simulink model "IEEE_39_case3"  (R2024b)
settings: Solver=ode3  StartTime=0  StopTime=40  FixedStep=Ts  MaxStep=1/60  RelTol=1e-3  AbsTol=1e-3  EnableMultiTasking=on
values from neighbouring files (symbols this model uses):
  c_f = c_f*Cb    [fun00_GFL_pu_2_normial.m]    (also in fun00_GFM_pu_2_normial.m)
  Dt = 0    [s02_case1.m]    (also in s02_case2.m; s03_case3.m; s03_case4.m; s03_case5.m)
  dw0_sm = 0    [s02_case1.m]    (also in s02_case2.m; s03_case3.m; s03_case4.m; s03_case5.m)
  Emax = 1.3    [s02_case1.m]    (also in s02_case2.m; s03_case3.m; s03_case4.m; s03_case5.m)
  Emin = 0.5    [s02_case1.m]    (also in s02_case2.m; s03_case3.m; s03_case4.m; s03_case5.m)
  Epss = 0.09    [s02_case1.m]    (also in s02_case2.m; s03_case3.m; s03_case4.m; s03_case5.m)
  fb = fn    (= 60)    [s02_case1.m]    (also in s02_case2.m; s03_case3.m; s03_case4.m; s03_case5.m)
  fn_sm = fn*ones(1,10)    [s02_case1.m]    (also in s02_case2.m; s03_case3.m; s03_case4.m; s03_case5.m)
  H_sm = [5,3.03,3.58,2.86,2.6,3.48,2.64,2.43,3.45,4.2]    [s02_case1.m]    (also in s02_case2.m; s03_case3.m; s03_case4.m; s03_case5.m)
  ia0_sm = 0    [s02_case1.m]    (also in s02_case2.m; s03_case3.m; s03_case4.m; s03_case5.m)
  ib0_sm = 0    [s02_case1.m]    (also in s02_case2.m; s03_case3.m; s03_case4.m; s03_case5.m)
  ic0_sm = 0    [s02_case1.m]    (also in s02_case2.m; s03_case3.m; s03_case4.m; s03_case5.m)
  Kd_sm = 0*ones(1,10)    [s02_case1.m]    (also in s02_case2.m; s03_case3.m; s03_case4.m; s03_case5.m)
  Ke = 1000    [s02_case1.m]    (also in s02_case2.m; s03_case3.m; s03_case4.m; s03_case5.m)
  ki_i = ki_i_pu*Vb_p_ph/Ib_p_ph    [fun00_GFL_pu_2_normial.m]    (also in fun00_GFM_pu_2_normial.m)
  ki_p = ki_p_pu/Sb*Ib_p_ph    [fun00_GFL_pu_2_normial.m]
  ki_pll = ki_pll/Vb_p_ph    [fun00_GFL_pu_2_normial.m]
  ki_q = ki_q_pu/Sb*Ib_p_ph    [fun00_GFL_pu_2_normial.m]
  kp_i = kp_i_pu*Vb_p_ph/Ib_p_ph    [fun00_GFL_pu_2_normial.m]    (also in fun00_GFM_pu_2_normial.m)
  kp_p = kp_p_pu/Sb*Ib_p_ph    [fun00_GFL_pu_2_normial.m]
  kp_pll = kp_pll/Vb_p_ph    [fun00_GFL_pu_2_normial.m]
  kp_q = kp_q_pu/Sb*Ib_p_ph    [fun00_GFL_pu_2_normial.m]
  Ks = 1    [s02_case1.m]    (also in s02_case2.m; s03_case3.m; s03_case4.m; s03_case5.m)
  l_f = l_f*Lb    [fun00_GFL_pu_2_normial.m]    (also in fun00_GFM_pu_2_normial.m)
  line = [     1	2	0.0035	0.0411	0.6987	0	100	345 ... (first row only)    [s02_case1.m]    (also in s02_case2.m; s03_case3.m; s03_case4.m; s03_case5.m)
  line_pu = line    [s02_case1.m]    (also in s02_case2.m; s03_case3.m; s03_case4.m; s03_case5.m)
  p = 1    [s02_case1.m]    (also in s02_case2.m; s03_case3.m; s03_case4.m; s03_case5.m)
  pha0_sm = 0    [s02_case1.m]    (also in s02_case2.m; s03_case3.m; s03_case4.m; s03_case5.m)
  phb0_sm = 0    [s02_case1.m]    (also in s02_case2.m; s03_case3.m; s03_case4.m; s03_case5.m)
  phc0_sm = 0    [s02_case1.m]    (also in s02_case2.m; s03_case3.m; s03_case4.m; s03_case5.m)
  Pn_sm = 1000*ones(1,num_gen)    [s02_case1.m]    (also in s02_case2.m; s03_case3.m; s03_case4.m; s03_case5.m)
  Pref_sm = [500 250 600 978 510 650 560 540 830 550]./Pn_sm    [s02_case1.m]    (also in s02_case2.m; s03_case3.m; s03_case4.m; s03_case5.m)
  pset = p_set_pu*Sb    [fun00_GFL_pu_2_normial.m]
  qset = q_set_pu*Sb    [fun00_GFL_pu_2_normial.m]
  R = 0.05    [s02_case1.m]    (also in s02_case2.m; s03_case3.m; s03_case4.m; s03_case5.m)
  r_f = r_f*Zb    [fun00_GFL_pu_2_normial.m]    (also in fun00_GFM_pu_2_normial.m)
  rs = 0.28    [s02_case1.m]    (also in s02_case2.m; s03_case3.m; s03_case4.m; s03_case5.m)
  Sb = 1000*10^6    (= 1000000000)    [s02_case1.m]    (also in s02_case2.m; s03_case3.m; s03_case4.m; s03_case5.m)
  T2 = 0.5    [s02_case1.m]    (also in s02_case2.m; s03_case3.m; s03_case4.m; s03_case5.m)
  T3 = 0.5    [s02_case1.m]    (also in s02_case2.m; s03_case3.m; s03_case4.m; s03_case5.m)
  t_gfl = 50    [s03_case3.m]    (also in s03_case4.m; s03_case5.m; s04_case6.m = 25; s04_case7.m = 25)
  t_gfm = 25    [s03_case3.m]    (also in s03_case4.m; s03_case5.m; s04_case6.m = 50; s04_case7.m = 50)
  t_s = 30    [s02_case1.m]    (also in s02_case2.m; s03_case3.m = 70; s03_case4.m = 70; s03_case5.m = 70)
  Te = 0.05    [s02_case1.m]    (also in s02_case2.m; s03_case3.m; s03_case4.m; s03_case5.m)
  Tfa = 3    [s02_case1.m]    (also in s02_case2.m; s03_case3.m; s03_case4.m; s03_case5.m)
  Tfb = 10    [s02_case1.m]    (also in s02_case2.m; s03_case3.m; s03_case4.m; s03_case5.m)
  theta0_sm = 0    [s02_case1.m]    (also in s02_case2.m; s03_case3.m; s03_case4.m; s03_case5.m)
  Ts = 1e-5    (= 1e-05)    [s02_case1.m]    (also in s02_case2.m; s03_case3.m; s03_case4.m; s03_case5.m)
  Ts1 = 0.76    [s02_case1.m]    (also in s02_case2.m; s03_case3.m; s03_case4.m; s03_case5.m)
  Ts2 = 0.1    [s02_case1.m]    (also in s02_case2.m; s03_case3.m; s03_case4.m; s03_case5.m)
  Ts3 = 0.76    [s02_case1.m]    (also in s02_case2.m; s03_case3.m; s03_case4.m; s03_case5.m)
  Ts4 = 0.1    [s02_case1.m]    (also in s02_case2.m; s03_case3.m; s03_case4.m; s03_case5.m)
  Ts5 = 10    [s02_case1.m]    (also in s02_case2.m; s03_case3.m; s03_case4.m; s03_case5.m)
  Un_sm = [345,22,22,22,22,22,22,22,345,22]    [s02_case1.m]    (also in s02_case2.m; s03_case3.m; s03_case4.m; s03_case5.m)
  Vb_gfm = 22*10^3    (= 22000)    [s02_case1.m]    (also in s02_case2.m; s03_case3.m; s03_case4.m; s03_case5.m)
  Vdc = 3*Vb_p_ph    [fun00_GFL_pu_2_normial.m]    (also in fun00_GFM_pu_2_normial.m)
  Vmax = 2    [s02_case1.m]    (also in s02_case2.m; s03_case3.m; s03_case4.m; s03_case5.m)
  Vmin = 0    [s02_case1.m]    (also in s02_case2.m; s03_case3.m; s03_case4.m; s03_case5.m)
  Vref_sm = 1*ones(1,10)    [s02_case1.m]    (also in s02_case2.m; s03_case3.m; s03_case4.m; s03_case5.m)
  w_b = fb*2*pi    [fun00_GFL_pu_2_normial.m]    (also in fun00_GFM_pu_2_normial.m; s02_case1.m = 376.991118431; s02_case2.m = 376.991118431; s03_case3.m = 376.991118431)
  wb = w_b    (= 376.991118431)    [s02_case1.m]    (also in s02_case2.m; s03_case3.m; s03_case4.m; s03_case5.m)
  xd = xd_t    (= 0.296)    [s02_case1.m]    (also in s02_case2.m; s03_case3.m; s03_case4.m; s03_case5.m)
undefined symbols (not defined in the file or in its folder): c_f_gfm, D1, D_p_gfm, D_p_gfm_s, D_q_gfm, Delta, DiscIntNeverNeededParam, Init, Init_GFL, J_gfm, Ka, Kf, ki_i_gfm, ki_pll_s, ki_vc_gfm, kp_i_gfm, kp_pll_s, kp_vc_gfm, l_f_gfm, P_set_gfm, Q_set_gfm, r_f_gfm, Ta, Tf, Vb, Vdc_gfm
libraries: spsThreePhaseVIMeasurementLib x76, spsabctodq0Lib x53, spsThreePhaseSeriesRLCBranchLib x52, slpidlib x50, spsThreePhaseParallelRLCLoadLib x20, spsThreePhaseTransformerTwoWindingsLib x12, spsdq0toabcLib x9, spsGroundLib x9, spsPowerPositiveSequenceLib x9, spsUniversalBridgeLib x9, spsDCVoltageSourceLib x9, spsFirstOrderFilterLib x1
(part 3 of 10)

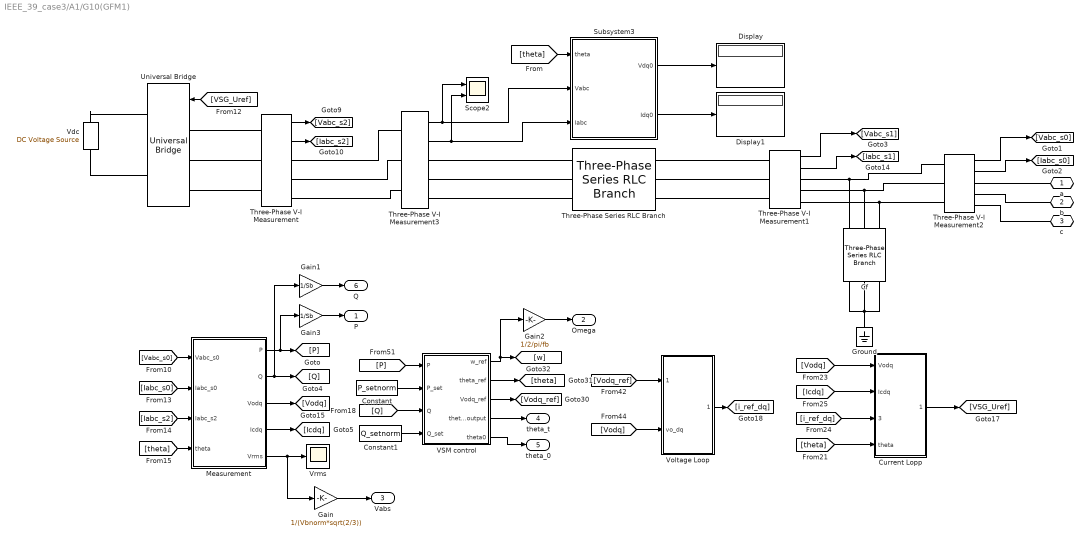
== system IEEE_39_case3/A1/G10(GFM1) ==
  Cf : spsThreePhaseSeriesRLCBranchLib/Three-Phase Series RLC Branch  LConnTagsString=A|B|C  RConnTagsString=A|B|C  BranchType=C  Resistance=0.1  Inductance=1e-3  Capacitance=RLCnorm(3)  Measurements=None
  Constant : Constant  Value=P_setnorm
  Constant1 : Constant  Value=Q_setnorm
  Current Lopp : Subsystem  mask{Current_P=Current_P, Current_I=Current_I}
      mask prompts: Current_P "Current Proportional Coefficient"; Current_I "Current Integral Coefficient"
  Display : Display
  Display1 : Display
  Gain : Gain  Gain=1/(Vbnorm*sqrt(2/3))
  Gain1 : Gain  Gain=1/Sb
  Gain2 : Gain  Gain=1/2/pi/fb
  Gain3 : Gain  Gain=1/Sb
  Ground : spsGroundLib/Ground  LConnTagsString=a
  Measurement : Subsystem
      mask DialogControl ParameterGroupVar Prompt: 参数
  Scope2 : Scope  NumInputPorts=2
  Subsystem3 : Subsystem
      mask DialogControl ParameterGroupVar Prompt: 参数
  Three-Phase Series RLC Branch : spsThreePhaseSeriesRLCBranchLib/Three-Phase Series RLC Branch  LConnTagsString=A|B|C  RConnTagsString=A|B|C  BranchType=RL  Resistance=RLCnorm(1)  Inductance=RLCnorm(2)  Capacitance=1e-6  Measurements=None
  Three-Phase V-I Measurement : spsThreePhaseVIMeasurementLib/Three-Phase V-I Measurement  VoltageMeasurement=phase-to-ground  SetLabelV=off  LabelV=Vabc_s2  Vpu=off  VpuLL=off  CurrentMeasurement=yes  SetLabelI=off  LabelI=Iabc_s2  Ipu=off  Pbase=Pnom  Vbase=Vnom  OutputType=Complex  PhasorSimulation=off  PSBequivalent=0
  Three-Phase V-I Measurement1 : spsThreePhaseVIMeasurementLib/Three-Phase V-I Measurement  VoltageMeasurement=phase-to-ground  SetLabelV=off  LabelV=Vabc_s1  Vpu=off  VpuLL=off  CurrentMeasurement=yes  SetLabelI=off  LabelI=Iabc_s1  Ipu=off  Pbase=Pnom  Vbase=Vnom  OutputType=Complex  PhasorSimulation=off  PSBequivalent=0
  Three-Phase V-I Measurement2 : spsThreePhaseVIMeasurementLib/Three-Phase V-I Measurement  VoltageMeasurement=phase-to-ground  SetLabelV=off  LabelV=Vabc_s0  Vpu=off  VpuLL=off  CurrentMeasurement=yes  SetLabelI=off  LabelI=Iabc_s0  Ipu=off  Pbase=Pnom  Vbase=Vnom  OutputType=Complex  PhasorSimulation=off  PSBequivalent=0
  Three-Phase V-I Measurement3 : spsThreePhaseVIMeasurementLib/Three-Phase V-I Measurement  VoltageMeasurement=phase-to-ground  SetLabelV=off  LabelV=Vabc_s2  Vpu=off  VpuLL=off  CurrentMeasurement=yes  SetLabelI=off  LabelI=Iabc_s2  Ipu=off  Pbase=Pnom  Vbase=Vnom  OutputType=Complex  PhasorSimulation=off  PSBequivalent=0
  Universal Bridge : spsUniversalBridgeLib/Universal Bridge  Arms=3  SnubberResistance=1e5  SnubberCapacitance=inf  Device=Average-model based VSC  Ron=1e-3  Lon=0  ForwardVoltages="[  0  0  ]"  ForwardVoltage=0  GTOparameters=[ 10e-6 , 20e-6 ]  IGBTparameters=[ 1e-6 , 2e-6 ]  Measurements=None  Measurements_2=None  converterType=Rectifier
  VSM control : Subsystem  mask{J=Jnorm, Dp=Dpnorm, Dq=Dqnorm}
      mask prompts: J "Inertia"; Dp "Damping"; Dq "Reactive Droop"
  Vdc : spsDCVoltageSourceLib/DC Voltage Source  Amplitude=Vdcnorm  Measurements=None
  Voltage Loop : Subsystem  mask{Voltage_P=Voltage_P, Voltage_I=Voltage_I}
      mask prompts: Voltage_P "Voltage Proportional Gain"; Voltage_I "Voltage Integral Gain"
  Vrms : Scope
  a : PMIOPort  Side=Right
  b : PMIOPort  Port=2  Side=Right
  c : PMIOPort  Port=3  Side=Right
  P : Outport
  Omega : Outport  Port=2
  Vabs : Outport  Port=3
  theta_t : Outport  Port=4
  theta_0 : Outport  Port=5
  Q : Outport  Port=6
  wires:
  [Vodq_ref] -> Voltage Loop/1(v_ref_dq)
  [Vodq] -> Voltage Loop/2(vo_dq)
  VSM control/2(theta_ref) -> [theta]
  Constant/1 -> VSM control/2(P_set)
  [P] -> VSM control/1(P)
  [Q] -> VSM control/3(Q)
  Three-Phase V-I Measurement1/2 -> [Iabc_s1]
  [VSG_Uref] -> Universal Bridge/1
  Subsystem3/1(Vdq0) -> Display/1
  Three-Phase V-I Measurement2/1 -> [Vabc_s0]
  Three-Phase V-I Measurement/2 -> [Iabc_s2]
  Three-Phase V-I Measurement3/2 -> Scope2/2, Subsystem3/3(Iabc)
  Subsystem3/2(Idq0) -> Display1/1
  Three-Phase V-I Measurement/1 -> [Vabc_s2]
  [theta] -> Subsystem3/1(theta)
  Three-Phase V-I Measurement2/2 -> [Iabc_s0]
  Three-Phase V-I Measurement3/1 -> Scope2/1, Subsystem3/2(Vabc)
  Three-Phase V-I Measurement1/1 -> [Vabc_s1]
  [Vabc_s0] -> Measurement/1(Vabc_s0)
  Measurement/5(Vrms) -> Gain/1, Vrms/1
  Measurement/2(Q) -> Gain1/1, [Q]
  Measurement/4(Icdq) -> [Icdq]
  Measurement/1(P) -> Gain3/1, [P]
  Measurement/3(Vodq) -> [Vodq]
  [theta] -> Measurement/4(theta)
  [Iabc_s2] -> Measurement/3(Iabc_s2)
  [Iabc_s0] -> Measurement/2(Iabc_s0)
  VSM control/3(Vodq_ref) -> [Vodq_ref]
  [Icdq] -> Current Lopp/2(Icdq)
  Current Lopp/1(VSG_Uref) -> [VSG_Uref]
  [Vodq] -> Current Lopp/1(Vodq)
  [theta] -> Current Lopp/4(theta)
  Voltage Loop/1(i_ref_dq) -> [i_ref_dq]
  [i_ref_dq] -> Current Lopp/3(i_ref_dq)
  Constant1/1 -> VSM control/4(Q_set)
  Gain/1 -> Vabs/1
  Gain3/1 -> P/1
  Gain2/1 -> Omega/1
  VSM control/1(w_ref) -> Gain2/1, [w]
  VSM control/4(theta_output) -> theta_t/1
  VSM control/5(theta0) -> theta_0/1
  Gain1/1 -> Q/1
  connections:
  Three-Phase V-I Measurement2/LConn1 -- Cf/LConn1 -- Three-Phase V-I Measurement1/RConn1
  Three-Phase V-I Measurement2/LConn2 -- Cf/LConn2 -- Three-Phase V-I Measurement1/RConn2
  Three-Phase V-I Measurement2/LConn3 -- Cf/LConn3 -- Three-Phase V-I Measurement1/RConn3
  Three-Phase V-I Measurement3/LConn1 -- Three-Phase V-I Measurement/RConn1
  Three-Phase V-I Measurement1/LConn3 -- Three-Phase Series RLC Branch/RConn3
  Three-Phase V-I Measurement2/RConn2 -- b/RConn1
  Three-Phase V-I Measurement/LConn3 -- Universal Bridge/LConn3
  Three-Phase V-I Measurement/LConn1 -- Universal Bridge/LConn1
  Vdc/RConn1 -- Universal Bridge/RConn1
  Three-Phase V-I Measurement2/RConn1 -- a/RConn1
  Three-Phase Series RLC Branch/LConn3 -- Three-Phase V-I Measurement3/RConn3
  Three-Phase V-I Measurement/LConn2 -- Universal Bridge/LConn2
  Three-Phase Series RLC Branch/LConn2 -- Three-Phase V-I Measurement3/RConn2
  Three-Phase V-I Measurement2/RConn3 -- c/RConn1
  Three-Phase V-I Measurement1/LConn1 -- Three-Phase Series RLC Branch/RConn1
  Three-Phase V-I Measurement3/RConn1 -- Three-Phase Series RLC Branch/LConn1
  Universal Bridge/RConn2 -- Vdc/LConn1
  Three-Phase V-I Measurement3/LConn3 -- Three-Phase V-I Measurement/RConn3
  Three-Phase V-I Measurement3/LConn2 -- Three-Phase V-I Measurement/RConn2
  Three-Phase V-I Measurement1/LConn2 -- Three-Phase Series RLC Branch/RConn2
  Cf/RConn3 -- Ground/LConn1 -- Cf/RConn2 -- Cf/RConn1

== system IEEE_39_case3/A1/G8(GFL4) ==
  Cf : spsThreePhaseSeriesRLCBranchLib/Three-Phase Series RLC Branch  LConnTagsString=A|B|C  RConnTagsString=A|B|C  BranchType=C  Resistance=0.1  Inductance=1e-3  Capacitance=RLC_Filter(3)  Measurements=None
  Constant : Constant  Value=Pref
  Constant1 : Constant  Value=Qref
  Display : Display
  Display1 : Display
  Gain : Gain  Gain=1/(Vnom*sqrt(2/3))
  Gain1 : Gain  Gain=1/Sb
  Gain2 : Gain  Gain=1/2/pi/fb
  Gain3 : Gain  Gain=1/Sb
  Ground : spsGroundLib/Ground  LConnTagsString=a
  Measurement : Subsystem
      mask DialogControl ParameterGroupVar Prompt: 参数
  PLL : Subsystem
      mask DialogControl ParameterGroupVar Prompt: 参数
  Subsystem3 : Subsystem
      mask DialogControl ParameterGroupVar Prompt: 参数
  Subsystem4 : Subsystem  mask{Voltage_P=Voltage_P, Voltage_I=Voltage_I, Current_P=Current_P, Current_I=Current_I, Power_P=Power_P, Power_I=Power_I, kf=kf}
      mask prompts: Voltage_P "Voltage Proportional Coefficient"; Voltage_I "Voltage Integral Coefficient"; Current_P "Current Proportional Coefficient"; Current_I "Current Integral Coefficient"; Power_P "Power Proportional Coefficient"; Power_I "Power Integral Coefficient"; kf "Feedforward Coeffcient"
      mask DialogControl ParameterGroupVar Prompt: Controller Parameter
  Three-Phase Series RLC Branch : spsThreePhaseSeriesRLCBranchLib/Three-Phase Series RLC Branch  LConnTagsString=A|B|C  RConnTagsString=A|B|C  BranchType=RL  Resistance=RLC_Filter(1)  Inductance=RLC_Filter(2)  Capacitance=1e-6  Measurements=None
  Three-Phase V-I Measurement : spsThreePhaseVIMeasurementLib/Three-Phase V-I Measurement  VoltageMeasurement=phase-to-ground  SetLabelV=off  LabelV=Vabc_s2  Vpu=off  VpuLL=off  CurrentMeasurement=yes  SetLabelI=off  LabelI=Iabc_s2  Ipu=off  Pbase=Pnom  Vbase=Vnom  OutputType=Complex  PhasorSimulation=off  PSBequivalent=0
  Three-Phase V-I Measurement1 : spsThreePhaseVIMeasurementLib/Three-Phase V-I Measurement  VoltageMeasurement=phase-to-ground  SetLabelV=off  LabelV=Vabc_s1  Vpu=off  VpuLL=off  CurrentMeasurement=yes  SetLabelI=off  LabelI=Iabc_s1  Ipu=off  Pbase=Pnom  Vbase=Vnom  OutputType=Complex  PhasorSimulation=off  PSBequivalent=0
  Three-Phase V-I Measurement2 : spsThreePhaseVIMeasurementLib/Three-Phase V-I Measurement  VoltageMeasurement=phase-to-ground  SetLabelV=off  LabelV=Vabc_s0  Vpu=off  VpuLL=off  CurrentMeasurement=yes  SetLabelI=off  LabelI=Iabc_s0  Ipu=off  Pbase=Pnom  Vbase=Vnom  OutputType=Complex  PhasorSimulation=off  PSBequivalent=0
  Three-Phase V-I Measurement3 : spsThreePhaseVIMeasurementLib/Three-Phase V-I Measurement  VoltageMeasurement=phase-to-ground  SetLabelV=off  LabelV=Vabc_s2  Vpu=off  VpuLL=off  CurrentMeasurement=yes  SetLabelI=off  LabelI=Iabc_s2  Ipu=off  Pbase=Pnom  Vbase=Vnom  OutputType=Complex  PhasorSimulation=off  PSBequivalent=0
  Universal Bridge : spsUniversalBridgeLib/Universal Bridge  Arms=3  SnubberResistance=1e5  SnubberCapacitance=inf  Device=Average-model based VSC  Ron=1e-3  Lon=0  ForwardVoltages="[  0  0  ]"  ForwardVoltage=0  GTOparameters=[ 10e-6 , 20e-6 ]  IGBTparameters=[ 1e-6 , 2e-6 ]  Measurements=None  Measurements_2=None  converterType=Rectifier
  Vdc : spsDCVoltageSourceLib/DC Voltage Source  Amplitude=Vdc_nom  Measurements=None
  Vrms : Scope
  a : PMIOPort  Side=Right
  b : PMIOPort  Port=2  Side=Right
  c : PMIOPort  Port=3  Side=Right
  P : Outport
  Omega : Outport  Port=2
  Vabs : Outport  Port=3
  theta_t : Outport  Port=4
  Q : Outport  Port=5
  theta_0 : Outport  Port=6
  wires:
  Measurement/5(Vrms) -> Gain/1, Vrms/1
  Measurement/2(Q) -> Gain1/1, [Q]
  Measurement/3(Vodq) -> [Vodq]
  Measurement/4(Icdq) -> [Icdq]
  [Vabc_s0] -> Measurement/1(Vabc_s0)
  [theta] -> Measurement/4(theta)
  [Iabc_s2] -> Measurement/3(Iabc_s2)
  [Iabc_s0] -> Measurement/2(Iabc_s0)
  [VSG_Uref] -> Universal Bridge/1
  [Vabc_s0] -> PLL/1(Vodq)
  Three-Phase V-I Measurement3/1 -> Subsystem3/1(Vabc)
  Three-Phase V-I Measurement3/2 -> Subsystem3/2(Iabc)
  Subsystem3/1(Vdq0) -> Display/1
  Subsystem3/2(Idq0) -> Display1/1
  PLL/2(theta) -> [theta]
  [Icdq] -> Subsystem4/2(Icdq)
  [Vodq] -> Subsystem4/1(Vodq)
  [theta] -> Subsystem4/3(theta)
  Subsystem4/1(VSG_Uref) -> [VSG_Uref]
  Three-Phase V-I Measurement/1 -> [Vabc_s2]
  Three-Phase V-I Measurement/2 -> [Iabc_s2]
  Three-Phase V-I Measurement2/1 -> [Vabc_s0]
  Three-Phase V-I Measurement2/2 -> [Iabc_s0]
  Three-Phase V-I Measurement1/2 -> [Iabc_s1]
  Three-Phase V-I Measurement1/1 -> [Vabc_s1]
  [P] -> Subsystem4/5(P)
  Constant/1 -> Subsystem4/4(pset)
  Constant1/1 -> Subsystem4/6(qset)
  [theta] -> Subsystem3/3(theta)
  Measurement/1(P) -> Gain3/1, [P]
  PLL/3(Omega) -> Gain2/1
  Gain/1 -> Vabs/1
  Gain2/1 -> Omega/1
  Gain3/1 -> P/1
  PLL/1(theta_GFL) -> theta_t/1
  Gain1/1 -> Q/1
  PLL/4(theta_0) -> theta_0/1
  [Q] -> Subsystem4/7(Q)
  connections:
  Three-Phase V-I Measurement2/LConn2 -- Cf/LConn2 -- Three-Phase V-I Measurement1/RConn2
  Three-Phase V-I Measurement2/LConn1 -- Cf/LConn1 -- Three-Phase V-I Measurement1/RConn1
  Three-Phase V-I Measurement2/LConn3 -- Cf/LConn3 -- Three-Phase V-I Measurement1/RConn3
  Three-Phase V-I Measurement1/LConn2 -- Three-Phase Series RLC Branch/RConn2
  Three-Phase V-I Measurement1/LConn1 -- Three-Phase Series RLC Branch/RConn1
  Universal Bridge/RConn2 -- Vdc/LConn1
  Vdc/RConn1 -- Universal Bridge/RConn1
  Three-Phase V-I Measurement/LConn3 -- Universal Bridge/LConn3
  Three-Phase V-I Measurement/LConn2 -- Universal Bridge/LConn2
  Three-Phase V-I Measurement/LConn1 -- Universal Bridge/LConn1
  Three-Phase V-I Measurement1/LConn3 -- Three-Phase Series RLC Branch/RConn3
  Three-Phase V-I Measurement2/RConn1 -- a/RConn1
  Three-Phase V-I Measurement2/RConn2 -- b/RConn1
  Three-Phase V-I Measurement2/RConn3 -- c/RConn1
  Three-Phase V-I Measurement3/RConn1 -- Three-Phase Series RLC Branch/LConn1
  Three-Phase Series RLC Branch/LConn2 -- Three-Phase V-I Measurement3/RConn2
  Three-Phase Series RLC Branch/LConn3 -- Three-Phase V-I Measurement3/RConn3
  Three-Phase V-I Measurement3/LConn1 -- Three-Phase V-I Measurement/RConn1
  Three-Phase V-I Measurement3/LConn2 -- Three-Phase V-I Measurement/RConn2
  Three-Phase V-I Measurement3/LConn3 -- Three-Phase V-I Measurement/RConn3
  Ground/LConn1 -- Cf/RConn2 -- Cf/RConn1 -- Cf/RConn3

== system IEEE_39_case3/A1/G9(GFL5) ==
  Cf : spsThreePhaseSeriesRLCBranchLib/Three-Phase Series RLC Branch  LConnTagsString=A|B|C  RConnTagsString=A|B|C  BranchType=C  Resistance=0.1  Inductance=1e-3  Capacitance=RLC_Filter(3)  Measurements=None
  Constant : Constant  Value=Pref
  Constant1 : Constant  Value=Qref
  Display : Display
  Display1 : Display
  Gain : Gain  Gain=1/(Vnom*sqrt(2/3))
  Gain1 : Gain  Gain=1/Sb
  Gain2 : Gain  Gain=1/2/pi/fb
  Gain3 : Gain  Gain=1/Sb
  Ground : spsGroundLib/Ground  LConnTagsString=a
  Measurement : Subsystem
      mask DialogControl ParameterGroupVar Prompt: 参数
  PLL : Subsystem
      mask DialogControl ParameterGroupVar Prompt: 参数
  Subsystem3 : Subsystem
      mask DialogControl ParameterGroupVar Prompt: 参数
  Subsystem4 : Subsystem  mask{Voltage_P=Voltage_P, Voltage_I=Voltage_I, Current_P=Current_P, Current_I=Current_I, Power_P=Power_P, Power_I=Power_I, kf=kf}
      mask prompts: Voltage_P "Voltage Proportional Coefficient"; Voltage_I "Voltage Integral Coefficient"; Current_P "Current Proportional Coefficient"; Current_I "Current Integral Coefficient"; Power_P "Power Proportional Coefficient"; Power_I "Power Integral Coefficient"; kf "Feedforward Coeffcient"
      mask DialogControl ParameterGroupVar Prompt: Controller Parameter
  Three-Phase Series RLC Branch : spsThreePhaseSeriesRLCBranchLib/Three-Phase Series RLC Branch  LConnTagsString=A|B|C  RConnTagsString=A|B|C  BranchType=RL  Resistance=RLC_Filter(1)  Inductance=RLC_Filter(2)  Capacitance=1e-6  Measurements=None
  Three-Phase V-I Measurement : spsThreePhaseVIMeasurementLib/Three-Phase V-I Measurement  VoltageMeasurement=phase-to-ground  SetLabelV=off  LabelV=Vabc_s2  Vpu=off  VpuLL=off  CurrentMeasurement=yes  SetLabelI=off  LabelI=Iabc_s2  Ipu=off  Pbase=Pnom  Vbase=Vnom  OutputType=Complex  PhasorSimulation=off  PSBequivalent=0
  Three-Phase V-I Measurement1 : spsThreePhaseVIMeasurementLib/Three-Phase V-I Measurement  VoltageMeasurement=phase-to-ground  SetLabelV=off  LabelV=Vabc_s1  Vpu=off  VpuLL=off  CurrentMeasurement=yes  SetLabelI=off  LabelI=Iabc_s1  Ipu=off  Pbase=Pnom  Vbase=Vnom  OutputType=Complex  PhasorSimulation=off  PSBequivalent=0
  Three-Phase V-I Measurement2 : spsThreePhaseVIMeasurementLib/Three-Phase V-I Measurement  VoltageMeasurement=phase-to-ground  SetLabelV=off  LabelV=Vabc_s0  Vpu=off  VpuLL=off  CurrentMeasurement=yes  SetLabelI=off  LabelI=Iabc_s0  Ipu=off  Pbase=Pnom  Vbase=Vnom  OutputType=Complex  PhasorSimulation=off  PSBequivalent=0
  Three-Phase V-I Measurement3 : spsThreePhaseVIMeasurementLib/Three-Phase V-I Measurement  VoltageMeasurement=phase-to-ground  SetLabelV=off  LabelV=Vabc_s2  Vpu=off  VpuLL=off  CurrentMeasurement=yes  SetLabelI=off  LabelI=Iabc_s2  Ipu=off  Pbase=Pnom  Vbase=Vnom  OutputType=Complex  PhasorSimulation=off  PSBequivalent=0
  Universal Bridge : spsUniversalBridgeLib/Universal Bridge  Arms=3  SnubberResistance=1e5  SnubberCapacitance=inf  Device=Average-model based VSC  Ron=1e-3  Lon=0  ForwardVoltages="[  0  0  ]"  ForwardVoltage=0  GTOparameters=[ 10e-6 , 20e-6 ]  IGBTparameters=[ 1e-6 , 2e-6 ]  Measurements=None  Measurements_2=None  converterType=Rectifier
  Vdc : spsDCVoltageSourceLib/DC Voltage Source  Amplitude=Vdc_nom  Measurements=None
  Vrms : Scope
  a : PMIOPort  Side=Right
  b : PMIOPort  Port=2  Side=Right
  c : PMIOPort  Port=3  Side=Right
  P : Outport
  Omega : Outport  Port=2
  Vabs : Outport  Port=3
  theta_t : Outport  Port=4
  Q : Outport  Port=5
  theta_0 : Outport  Port=6
  wires:
  Measurement/5(Vrms) -> Gain/1, Vrms/1
  Measurement/2(Q) -> Gain1/1, [Q]
  Measurement/3(Vodq) -> [Vodq]
  Measurement/4(Icdq) -> [Icdq]
  [Vabc_s0] -> Measurement/1(Vabc_s0)
  [theta] -> Measurement/4(theta)
  [Iabc_s2] -> Measurement/3(Iabc_s2)
  [Iabc_s0] -> Measurement/2(Iabc_s0)
  [VSG_Uref] -> Universal Bridge/1
  [Vabc_s0] -> PLL/1(Vodq)
  Three-Phase V-I Measurement3/1 -> Subsystem3/1(Vabc)
  Three-Phase V-I Measurement3/2 -> Subsystem3/2(Iabc)
  Subsystem3/1(Vdq0) -> Display/1
  Subsystem3/2(Idq0) -> Display1/1
  PLL/2(theta) -> [theta]
  [Icdq] -> Subsystem4/2(Icdq)
  [Vodq] -> Subsystem4/1(Vodq)
  [theta] -> Subsystem4/3(theta)
  Subsystem4/1(VSG_Uref) -> [VSG_Uref]
  Three-Phase V-I Measurement/1 -> [Vabc_s2]
  Three-Phase V-I Measurement/2 -> [Iabc_s2]
  Three-Phase V-I Measurement2/1 -> [Vabc_s0]
  Three-Phase V-I Measurement2/2 -> [Iabc_s0]
  Three-Phase V-I Measurement1/2 -> [Iabc_s1]
  Three-Phase V-I Measurement1/1 -> [Vabc_s1]
  [P] -> Subsystem4/5(P)
  Constant/1 -> Subsystem4/4(pset)
  Constant1/1 -> Subsystem4/6(qset)
  [theta] -> Subsystem3/3(theta)
  Measurement/1(P) -> Gain3/1, [P]
  PLL/3(Omega) -> Gain2/1
  Gain/1 -> Vabs/1
  Gain2/1 -> Omega/1
  Gain3/1 -> P/1
  PLL/1(theta_GFL) -> theta_t/1
  Gain1/1 -> Q/1
  PLL/4(theta_0) -> theta_0/1
  [Q] -> Subsystem4/7(Q)
  connections:
  Three-Phase V-I Measurement2/LConn2 -- Cf/LConn2 -- Three-Phase V-I Measurement1/RConn2
  Three-Phase V-I Measurement2/LConn1 -- Cf/LConn1 -- Three-Phase V-I Measurement1/RConn1
  Three-Phase V-I Measurement2/LConn3 -- Cf/LConn3 -- Three-Phase V-I Measurement1/RConn3
  Three-Phase V-I Measurement1/LConn2 -- Three-Phase Series RLC Branch/RConn2
  Three-Phase V-I Measurement1/LConn1 -- Three-Phase Series RLC Branch/RConn1
  Universal Bridge/RConn2 -- Vdc/LConn1
  Vdc/RConn1 -- Universal Bridge/RConn1
  Three-Phase V-I Measurement/LConn3 -- Universal Bridge/LConn3
  Three-Phase V-I Measurement/LConn2 -- Universal Bridge/LConn2
  Three-Phase V-I Measurement/LConn1 -- Universal Bridge/LConn1
  Three-Phase V-I Measurement1/LConn3 -- Three-Phase Series RLC Branch/RConn3
  Three-Phase V-I Measurement2/RConn1 -- a/RConn1
  Three-Phase V-I Measurement2/RConn2 -- b/RConn1
  Three-Phase V-I Measurement2/RConn3 -- c/RConn1
  Three-Phase V-I Measurement3/RConn1 -- Three-Phase Series RLC Branch/LConn1
  Three-Phase Series RLC Branch/LConn2 -- Three-Phase V-I Measurement3/RConn2
  Three-Phase Series RLC Branch/LConn3 -- Three-Phase V-I Measurement3/RConn3
  Three-Phase V-I Measurement3/LConn1 -- Three-Phase V-I Measurement/RConn1
  Three-Phase V-I Measurement3/LConn2 -- Three-Phase V-I Measurement/RConn2
  Three-Phase V-I Measurement3/LConn3 -- Three-Phase V-I Measurement/RConn3
  Ground/LConn1 -- Cf/RConn2 -- Cf/RConn1 -- Cf/RConn3

== system IEEE_39_case3/A2/G1(GFL1) ==
  Cf : spsThreePhaseSeriesRLCBranchLib/Three-Phase Series RLC Branch  LConnTagsString=A|B|C  RConnTagsString=A|B|C  BranchType=C  Resistance=0.1  Inductance=1e-3  Capacitance=RLC_Filter(3)  Measurements=None
  Constant : Constant  Value=Pref
  Constant1 : Constant  Value=Qref
  Display : Display
  Display1 : Display
  Gain : Gain  Gain=1/(Vnom*sqrt(2/3))
  Gain1 : Gain  Gain=1/Sb
  Gain2 : Gain  Gain=1/2/pi/fb
  Gain3 : Gain  Gain=1/Sb
  Ground : spsGroundLib/Ground  LConnTagsString=a
  Measurement : Subsystem
      mask DialogControl ParameterGroupVar Prompt: 参数
  PLL : Subsystem
      mask DialogControl ParameterGroupVar Prompt: 参数
  Subsystem3 : Subsystem
      mask DialogControl ParameterGroupVar Prompt: 参数
  Subsystem4 : Subsystem  mask{Voltage_P=Voltage_P, Voltage_I=Voltage_I, Current_P=Current_P, Current_I=Current_I, Power_P=Power_P, Power_I=Power_I, kf=kf}
      mask prompts: Voltage_P "Voltage Proportional Coefficient"; Voltage_I "Voltage Integral Coefficient"; Current_P "Current Proportional Coefficient"; Current_I "Current Integral Coefficient"; Power_P "Power Proportional Coefficient"; Power_I "Power Integral Coefficient"; kf "Feedforward Coeffcient"
      mask DialogControl ParameterGroupVar Prompt: Controller Parameter
  Three-Phase Series RLC Branch : spsThreePhaseSeriesRLCBranchLib/Three-Phase Series RLC Branch  LConnTagsString=A|B|C  RConnTagsString=A|B|C  BranchType=RL  Resistance=RLC_Filter(1)  Inductance=RLC_Filter(2)  Capacitance=1e-6  Measurements=None
  Three-Phase V-I Measurement : spsThreePhaseVIMeasurementLib/Three-Phase V-I Measurement  VoltageMeasurement=phase-to-ground  SetLabelV=off  LabelV=Vabc_s2  Vpu=off  VpuLL=off  CurrentMeasurement=yes  SetLabelI=off  LabelI=Iabc_s2  Ipu=off  Pbase=Pnom  Vbase=Vnom  OutputType=Complex  PhasorSimulation=off  PSBequivalent=0
  Three-Phase V-I Measurement1 : spsThreePhaseVIMeasurementLib/Three-Phase V-I Measurement  VoltageMeasurement=phase-to-ground  SetLabelV=off  LabelV=Vabc_s1  Vpu=off  VpuLL=off  CurrentMeasurement=yes  SetLabelI=off  LabelI=Iabc_s1  Ipu=off  Pbase=Pnom  Vbase=Vnom  OutputType=Complex  PhasorSimulation=off  PSBequivalent=0
  Three-Phase V-I Measurement2 : spsThreePhaseVIMeasurementLib/Three-Phase V-I Measurement  VoltageMeasurement=phase-to-ground  SetLabelV=off  LabelV=Vabc_s0  Vpu=off  VpuLL=off  CurrentMeasurement=yes  SetLabelI=off  LabelI=Iabc_s0  Ipu=off  Pbase=Pnom  Vbase=Vnom  OutputType=Complex  PhasorSimulation=off  PSBequivalent=0
  Three-Phase V-I Measurement3 : spsThreePhaseVIMeasurementLib/Three-Phase V-I Measurement  VoltageMeasurement=phase-to-ground  SetLabelV=off  LabelV=Vabc_s2  Vpu=off  VpuLL=off  CurrentMeasurement=yes  SetLabelI=off  LabelI=Iabc_s2  Ipu=off  Pbase=Pnom  Vbase=Vnom  OutputType=Complex  PhasorSimulation=off  PSBequivalent=0
  Universal Bridge : spsUniversalBridgeLib/Universal Bridge  Arms=3  SnubberResistance=1e5  SnubberCapacitance=inf  Device=Average-model based VSC  Ron=1e-3  Lon=0  ForwardVoltages="[  0  0  ]"  ForwardVoltage=0  GTOparameters=[ 10e-6 , 20e-6 ]  IGBTparameters=[ 1e-6 , 2e-6 ]  Measurements=None  Measurements_2=None  converterType=Rectifier
  Vdc : spsDCVoltageSourceLib/DC Voltage Source  Amplitude=Vdc_nom  Measurements=None
  Vrms : Scope
  a : PMIOPort  Side=Right
  b : PMIOPort  Port=2  Side=Right
  c : PMIOPort  Port=3  Side=Right
  P : Outport
  Omega : Outport  Port=2
  Vabs : Outport  Port=3
  theta_t : Outport  Port=4
  Q : Outport  Port=5
  theta_0 : Outport  Port=6
  wires:
  Measurement/5(Vrms) -> Gain/1, Vrms/1
  Measurement/2(Q) -> Gain1/1, [Q]
  Measurement/3(Vodq) -> [Vodq]
  Measurement/4(Icdq) -> [Icdq]
  [Vabc_s0] -> Measurement/1(Vabc_s0)
  [theta] -> Measurement/4(theta)
  [Iabc_s2] -> Measurement/3(Iabc_s2)
  [Iabc_s0] -> Measurement/2(Iabc_s0)
  [VSG_Uref] -> Universal Bridge/1
  [Vabc_s0] -> PLL/1(Vodq)
  Three-Phase V-I Measurement3/1 -> Subsystem3/1(Vabc)
  Three-Phase V-I Measurement3/2 -> Subsystem3/2(Iabc)
  Subsystem3/1(Vdq0) -> Display/1
  Subsystem3/2(Idq0) -> Display1/1
  PLL/2(theta) -> [theta]
  [Icdq] -> Subsystem4/2(Icdq)
  [Vodq] -> Subsystem4/1(Vodq)
  [theta] -> Subsystem4/3(theta)
  Subsystem4/1(VSG_Uref) -> [VSG_Uref]
  Three-Phase V-I Measurement/1 -> [Vabc_s2]
  Three-Phase V-I Measurement/2 -> [Iabc_s2]
  Three-Phase V-I Measurement2/1 -> [Vabc_s0]
  Three-Phase V-I Measurement2/2 -> [Iabc_s0]
  Three-Phase V-I Measurement1/2 -> [Iabc_s1]
  Three-Phase V-I Measurement1/1 -> [Vabc_s1]
  [P] -> Subsystem4/5(P)
  Constant/1 -> Subsystem4/4(pset)
  Constant1/1 -> Subsystem4/6(qset)
  [theta] -> Subsystem3/3(theta)
  Measurement/1(P) -> Gain3/1, [P]
  PLL/3(Omega) -> Gain2/1
  Gain/1 -> Vabs/1
  Gain2/1 -> Omega/1
  Gain3/1 -> P/1
  PLL/1(theta_GFL) -> theta_t/1
  Gain1/1 -> Q/1
  PLL/4(theta_0) -> theta_0/1
  [Q] -> Subsystem4/7(Q)
  connections:
  Three-Phase V-I Measurement2/LConn2 -- Cf/LConn2 -- Three-Phase V-I Measurement1/RConn2
  Three-Phase V-I Measurement2/LConn1 -- Cf/LConn1 -- Three-Phase V-I Measurement1/RConn1
  Three-Phase V-I Measurement2/LConn3 -- Cf/LConn3 -- Three-Phase V-I Measurement1/RConn3
  Three-Phase V-I Measurement1/LConn2 -- Three-Phase Series RLC Branch/RConn2
  Three-Phase V-I Measurement1/LConn1 -- Three-Phase Series RLC Branch/RConn1
  Universal Bridge/RConn2 -- Vdc/LConn1
  Vdc/RConn1 -- Universal Bridge/RConn1
  Three-Phase V-I Measurement/LConn3 -- Universal Bridge/LConn3
  Three-Phase V-I Measurement/LConn2 -- Universal Bridge/LConn2
  Three-Phase V-I Measurement/LConn1 -- Universal Bridge/LConn1
  Three-Phase V-I Measurement1/LConn3 -- Three-Phase Series RLC Branch/RConn3
  Three-Phase V-I Measurement2/RConn1 -- a/RConn1
  Three-Phase V-I Measurement2/RConn2 -- b/RConn1
  Three-Phase V-I Measurement2/RConn3 -- c/RConn1
  Three-Phase V-I Measurement3/RConn1 -- Three-Phase Series RLC Branch/LConn1
  Three-Phase Series RLC Branch/LConn2 -- Three-Phase V-I Measurement3/RConn2
  Three-Phase Series RLC Branch/LConn3 -- Three-Phase V-I Measurement3/RConn3
  Three-Phase V-I Measurement3/LConn1 -- Three-Phase V-I Measurement/RConn1
  Three-Phase V-I Measurement3/LConn2 -- Three-Phase V-I Measurement/RConn2
  Three-Phase V-I Measurement3/LConn3 -- Three-Phase V-I Measurement/RConn3
  Ground/LConn1 -- Cf/RConn2 -- Cf/RConn1 -- Cf/RConn3

== system IEEE_39_case3/A2/G2(GFL2) ==
  Cf : spsThreePhaseSeriesRLCBranchLib/Three-Phase Series RLC Branch  LConnTagsString=A|B|C  RConnTagsString=A|B|C  BranchType=C  Resistance=0.1  Inductance=1e-3  Capacitance=RLC_Filter(3)  Measurements=None
  Constant : Constant  Value=Pref
  Constant1 : Constant  Value=Qref
  Display : Display
  Display1 : Display
  Gain : Gain  Gain=1/(Vnom*sqrt(2/3))
  Gain1 : Gain  Gain=1/Sb
  Gain2 : Gain  Gain=1/2/pi/fb
  Gain3 : Gain  Gain=1/Sb
  Ground : spsGroundLib/Ground  LConnTagsString=a
  Measurement : Subsystem
      mask DialogControl ParameterGroupVar Prompt: 参数
  PLL : Subsystem
      mask DialogControl ParameterGroupVar Prompt: 参数
  Subsystem3 : Subsystem
      mask DialogControl ParameterGroupVar Prompt: 参数
  Subsystem4 : Subsystem  mask{Voltage_P=Voltage_P, Voltage_I=Voltage_I, Current_P=Current_P, Current_I=Current_I, Power_P=Power_P, Power_I=Power_I, kf=kf}
      mask prompts: Voltage_P "Voltage Proportional Coefficient"; Voltage_I "Voltage Integral Coefficient"; Current_P "Current Proportional Coefficient"; Current_I "Current Integral Coefficient"; Power_P "Power Proportional Coefficient"; Power_I "Power Integral Coefficient"; kf "Feedforward Coeffcient"
      mask DialogControl ParameterGroupVar Prompt: Controller Parameter
  Three-Phase Series RLC Branch : spsThreePhaseSeriesRLCBranchLib/Three-Phase Series RLC Branch  LConnTagsString=A|B|C  RConnTagsString=A|B|C  BranchType=RL  Resistance=RLC_Filter(1)  Inductance=RLC_Filter(2)  Capacitance=1e-6  Measurements=None
  Three-Phase V-I Measurement : spsThreePhaseVIMeasurementLib/Three-Phase V-I Measurement  VoltageMeasurement=phase-to-ground  SetLabelV=off  LabelV=Vabc_s2  Vpu=off  VpuLL=off  CurrentMeasurement=yes  SetLabelI=off  LabelI=Iabc_s2  Ipu=off  Pbase=Pnom  Vbase=Vnom  OutputType=Complex  PhasorSimulation=off  PSBequivalent=0
  Three-Phase V-I Measurement1 : spsThreePhaseVIMeasurementLib/Three-Phase V-I Measurement  VoltageMeasurement=phase-to-ground  SetLabelV=off  LabelV=Vabc_s1  Vpu=off  VpuLL=off  CurrentMeasurement=yes  SetLabelI=off  LabelI=Iabc_s1  Ipu=off  Pbase=Pnom  Vbase=Vnom  OutputType=Complex  PhasorSimulation=off  PSBequivalent=0
  Three-Phase V-I Measurement2 : spsThreePhaseVIMeasurementLib/Three-Phase V-I Measurement  VoltageMeasurement=phase-to-ground  SetLabelV=off  LabelV=Vabc_s0  Vpu=off  VpuLL=off  CurrentMeasurement=yes  SetLabelI=off  LabelI=Iabc_s0  Ipu=off  Pbase=Pnom  Vbase=Vnom  OutputType=Complex  PhasorSimulation=off  PSBequivalent=0
  Three-Phase V-I Measurement3 : spsThreePhaseVIMeasurementLib/Three-Phase V-I Measurement  VoltageMeasurement=phase-to-ground  SetLabelV=off  LabelV=Vabc_s2  Vpu=off  VpuLL=off  CurrentMeasurement=yes  SetLabelI=off  LabelI=Iabc_s2  Ipu=off  Pbase=Pnom  Vbase=Vnom  OutputType=Complex  PhasorSimulation=off  PSBequivalent=0
  Universal Bridge : spsUniversalBridgeLib/Universal Bridge  Arms=3  SnubberResistance=1e5  SnubberCapacitance=inf  Device=Average-model based VSC  Ron=1e-3  Lon=0  ForwardVoltages="[  0  0  ]"  ForwardVoltage=0  GTOparameters=[ 10e-6 , 20e-6 ]  IGBTparameters=[ 1e-6 , 2e-6 ]  Measurements=None  Measurements_2=None  converterType=Rectifier
  Vdc : spsDCVoltageSourceLib/DC Voltage Source  Amplitude=Vdc_nom  Measurements=None
  Vrms : Scope
  a : PMIOPort  Side=Right
  b : PMIOPort  Port=2  Side=Right
  c : PMIOPort  Port=3  Side=Right
  P : Outport
  Omega : Outport  Port=2
  Vabs : Outport  Port=3
  theta_t : Outport  Port=4
  Q : Outport  Port=5
  theta_0 : Outport  Port=6
  wires:
  Measurement/5(Vrms) -> Gain/1, Vrms/1
  Measurement/2(Q) -> Gain1/1, [Q]
  Measurement/3(Vodq) -> [Vodq]
  Measurement/4(Icdq) -> [Icdq]
  [Vabc_s0] -> Measurement/1(Vabc_s0)
  [theta] -> Measurement/4(theta)
  [Iabc_s2] -> Measurement/3(Iabc_s2)
  [Iabc_s0] -> Measurement/2(Iabc_s0)
  [VSG_Uref] -> Universal Bridge/1
  [Vabc_s0] -> PLL/1(Vodq)
  Three-Phase V-I Measurement3/1 -> Subsystem3/1(Vabc)
  Three-Phase V-I Measurement3/2 -> Subsystem3/2(Iabc)
  Subsystem3/1(Vdq0) -> Display/1
  Subsystem3/2(Idq0) -> Display1/1
  PLL/2(theta) -> [theta]
  [Icdq] -> Subsystem4/2(Icdq)
  [Vodq] -> Subsystem4/1(Vodq)
  [theta] -> Subsystem4/3(theta)
  Subsystem4/1(VSG_Uref) -> [VSG_Uref]
  Three-Phase V-I Measurement/1 -> [Vabc_s2]
  Three-Phase V-I Measurement/2 -> [Iabc_s2]
  Three-Phase V-I Measurement2/1 -> [Vabc_s0]
  Three-Phase V-I Measurement2/2 -> [Iabc_s0]
  Three-Phase V-I Measurement1/2 -> [Iabc_s1]
  Three-Phase V-I Measurement1/1 -> [Vabc_s1]
  [P] -> Subsystem4/5(P)
  Constant/1 -> Subsystem4/4(pset)
  Constant1/1 -> Subsystem4/6(qset)
  [theta] -> Subsystem3/3(theta)
  Measurement/1(P) -> Gain3/1, [P]
  PLL/3(Omega) -> Gain2/1
  Gain/1 -> Vabs/1
  Gain2/1 -> Omega/1
  Gain3/1 -> P/1
  PLL/1(theta_GFL) -> theta_t/1
  Gain1/1 -> Q/1
  PLL/4(theta_0) -> theta_0/1
  [Q] -> Subsystem4/7(Q)
  connections:
  Three-Phase V-I Measurement2/LConn2 -- Cf/LConn2 -- Three-Phase V-I Measurement1/RConn2
  Three-Phase V-I Measurement2/LConn1 -- Cf/LConn1 -- Three-Phase V-I Measurement1/RConn1
  Three-Phase V-I Measurement2/LConn3 -- Cf/LConn3 -- Three-Phase V-I Measurement1/RConn3
  Three-Phase V-I Measurement1/LConn2 -- Three-Phase Series RLC Branch/RConn2
  Three-Phase V-I Measurement1/LConn1 -- Three-Phase Series RLC Branch/RConn1
  Universal Bridge/RConn2 -- Vdc/LConn1
  Vdc/RConn1 -- Universal Bridge/RConn1
  Three-Phase V-I Measurement/LConn3 -- Universal Bridge/LConn3
  Three-Phase V-I Measurement/LConn2 -- Universal Bridge/LConn2
  Three-Phase V-I Measurement/LConn1 -- Universal Bridge/LConn1
  Three-Phase V-I Measurement1/LConn3 -- Three-Phase Series RLC Branch/RConn3
  Three-Phase V-I Measurement2/RConn1 -- a/RConn1
  Three-Phase V-I Measurement2/RConn2 -- b/RConn1
  Three-Phase V-I Measurement2/RConn3 -- c/RConn1
  Three-Phase V-I Measurement3/RConn1 -- Three-Phase Series RLC Branch/LConn1
  Three-Phase Series RLC Branch/LConn2 -- Three-Phase V-I Measurement3/RConn2
  Three-Phase Series RLC Branch/LConn3 -- Three-Phase V-I Measurement3/RConn3
  Three-Phase V-I Measurement3/LConn1 -- Three-Phase V-I Measurement/RConn1
  Three-Phase V-I Measurement3/LConn2 -- Three-Phase V-I Measurement/RConn2
  Three-Phase V-I Measurement3/LConn3 -- Three-Phase V-I Measurement/RConn3
  Ground/LConn1 -- Cf/RConn2 -- Cf/RConn1 -- Cf/RConn3

== system IEEE_39_case3/A2/G3(GFL7) ==
  Cf : spsThreePhaseSeriesRLCBranchLib/Three-Phase Series RLC Branch  LConnTagsString=A|B|C  RConnTagsString=A|B|C  BranchType=C  Resistance=0.1  Inductance=1e-3  Capacitance=RLC_Filter(3)  Measurements=None
  Constant : Constant  Value=Pref
  Constant1 : Constant  Value=Qref
  Display : Display
  Display1 : Display
  Gain : Gain  Gain=1/(Vnom*sqrt(2/3))
  Gain1 : Gain  Gain=1/Sb
  Gain2 : Gain  Gain=1/2/pi/fb
  Gain3 : Gain  Gain=1/Sb
  Ground : spsGroundLib/Ground  LConnTagsString=a
  Measurement : Subsystem
      mask DialogControl ParameterGroupVar Prompt: 参数
  PLL : Subsystem
      mask DialogControl ParameterGroupVar Prompt: 参数
  Subsystem3 : Subsystem
      mask DialogControl ParameterGroupVar Prompt: 参数
  Subsystem4 : Subsystem  mask{Voltage_P=Voltage_P, Voltage_I=Voltage_I, Current_P=Current_P, Current_I=Current_I, Power_P=Power_P, Power_I=Power_I, kf=kf}
      mask prompts: Voltage_P "Voltage Proportional Coefficient"; Voltage_I "Voltage Integral Coefficient"; Current_P "Current Proportional Coefficient"; Current_I "Current Integral Coefficient"; Power_P "Power Proportional Coefficient"; Power_I "Power Integral Coefficient"; kf "Feedforward Coeffcient"
      mask DialogControl ParameterGroupVar Prompt: Controller Parameter
  Three-Phase Series RLC Branch : spsThreePhaseSeriesRLCBranchLib/Three-Phase Series RLC Branch  LConnTagsString=A|B|C  RConnTagsString=A|B|C  BranchType=RL  Resistance=RLC_Filter(1)  Inductance=RLC_Filter(2)  Capacitance=1e-6  Measurements=None
  Three-Phase V-I Measurement : spsThreePhaseVIMeasurementLib/Three-Phase V-I Measurement  VoltageMeasurement=phase-to-ground  SetLabelV=off  LabelV=Vabc_s2  Vpu=off  VpuLL=off  CurrentMeasurement=yes  SetLabelI=off  LabelI=Iabc_s2  Ipu=off  Pbase=Pnom  Vbase=Vnom  OutputType=Complex  PhasorSimulation=off  PSBequivalent=0
  Three-Phase V-I Measurement1 : spsThreePhaseVIMeasurementLib/Three-Phase V-I Measurement  VoltageMeasurement=phase-to-ground  SetLabelV=off  LabelV=Vabc_s1  Vpu=off  VpuLL=off  CurrentMeasurement=yes  SetLabelI=off  LabelI=Iabc_s1  Ipu=off  Pbase=Pnom  Vbase=Vnom  OutputType=Complex  PhasorSimulation=off  PSBequivalent=0
  Three-Phase V-I Measurement2 : spsThreePhaseVIMeasurementLib/Three-Phase V-I Measurement  VoltageMeasurement=phase-to-ground  SetLabelV=off  LabelV=Vabc_s0  Vpu=off  VpuLL=off  CurrentMeasurement=yes  SetLabelI=off  LabelI=Iabc_s0  Ipu=off  Pbase=Pnom  Vbase=Vnom  OutputType=Complex  PhasorSimulation=off  PSBequivalent=0
  Three-Phase V-I Measurement3 : spsThreePhaseVIMeasurementLib/Three-Phase V-I Measurement  VoltageMeasurement=phase-to-ground  SetLabelV=off  LabelV=Vabc_s2  Vpu=off  VpuLL=off  CurrentMeasurement=yes  SetLabelI=off  LabelI=Iabc_s2  Ipu=off  Pbase=Pnom  Vbase=Vnom  OutputType=Complex  PhasorSimulation=off  PSBequivalent=0
  Universal Bridge : spsUniversalBridgeLib/Universal Bridge  Arms=3  SnubberResistance=1e5  SnubberCapacitance=inf  Device=Average-model based VSC  Ron=1e-3  Lon=0  ForwardVoltages="[  0  0  ]"  ForwardVoltage=0  GTOparameters=[ 10e-6 , 20e-6 ]  IGBTparameters=[ 1e-6 , 2e-6 ]  Measurements=None  Measurements_2=None  converterType=Rectifier
  Vdc : spsDCVoltageSourceLib/DC Voltage Source  Amplitude=Vdc_nom  Measurements=None
  Vrms : Scope
  a : PMIOPort  Side=Right
  b : PMIOPort  Port=2  Side=Right
  c : PMIOPort  Port=3  Side=Right
  P : Outport
  Omega : Outport  Port=2
  Vabs : Outport  Port=3
  theta_t : Outport  Port=4
  Q : Outport  Port=5
  theta_0 : Outport  Port=6
  wires:
  Measurement/5(Vrms) -> Gain/1, Vrms/1
  Measurement/2(Q) -> Gain1/1, [Q]
  Measurement/3(Vodq) -> [Vodq]
  Measurement/4(Icdq) -> [Icdq]
  [Vabc_s0] -> Measurement/1(Vabc_s0)
  [theta] -> Measurement/4(theta)
  [Iabc_s2] -> Measurement/3(Iabc_s2)
  [Iabc_s0] -> Measurement/2(Iabc_s0)
  [VSG_Uref] -> Universal Bridge/1
  [Vabc_s0] -> PLL/1(Vodq)
  Three-Phase V-I Measurement3/1 -> Subsystem3/1(Vabc)
  Three-Phase V-I Measurement3/2 -> Subsystem3/2(Iabc)
  Subsystem3/1(Vdq0) -> Display/1
  Subsystem3/2(Idq0) -> Display1/1
  PLL/2(theta) -> [theta]
  [Icdq] -> Subsystem4/2(Icdq)
  [Vodq] -> Subsystem4/1(Vodq)
  [theta] -> Subsystem4/3(theta)
  Subsystem4/1(VSG_Uref) -> [VSG_Uref]
  Three-Phase V-I Measurement/1 -> [Vabc_s2]
  Three-Phase V-I Measurement/2 -> [Iabc_s2]
  Three-Phase V-I Measurement2/1 -> [Vabc_s0]
  Three-Phase V-I Measurement2/2 -> [Iabc_s0]
  Three-Phase V-I Measurement1/2 -> [Iabc_s1]
  Three-Phase V-I Measurement1/1 -> [Vabc_s1]
  [P] -> Subsystem4/5(P)
  Constant/1 -> Subsystem4/4(pset)
  Constant1/1 -> Subsystem4/6(qset)
  [theta] -> Subsystem3/3(theta)
  Measurement/1(P) -> Gain3/1, [P]
  PLL/3(Omega) -> Gain2/1
  Gain/1 -> Vabs/1
  Gain2/1 -> Omega/1
  Gain3/1 -> P/1
  PLL/1(theta_GFL) -> theta_t/1
  Gain1/1 -> Q/1
  PLL/4(theta_0) -> theta_0/1
  [Q] -> Subsystem4/7(Q)
  connections:
  Three-Phase V-I Measurement2/LConn2 -- Cf/LConn2 -- Three-Phase V-I Measurement1/RConn2
  Three-Phase V-I Measurement2/LConn1 -- Cf/LConn1 -- Three-Phase V-I Measurement1/RConn1
  Three-Phase V-I Measurement2/LConn3 -- Cf/LConn3 -- Three-Phase V-I Measurement1/RConn3
  Three-Phase V-I Measurement1/LConn2 -- Three-Phase Series RLC Branch/RConn2
  Three-Phase V-I Measurement1/LConn1 -- Three-Phase Series RLC Branch/RConn1
  Universal Bridge/RConn2 -- Vdc/LConn1
  Vdc/RConn1 -- Universal Bridge/RConn1
  Three-Phase V-I Measurement/LConn3 -- Universal Bridge/LConn3
  Three-Phase V-I Measurement/LConn2 -- Universal Bridge/LConn2
  Three-Phase V-I Measurement/LConn1 -- Universal Bridge/LConn1
  Three-Phase V-I Measurement1/LConn3 -- Three-Phase Series RLC Branch/RConn3
  Three-Phase V-I Measurement2/RConn1 -- a/RConn1
  Three-Phase V-I Measurement2/RConn2 -- b/RConn1
  Three-Phase V-I Measurement2/RConn3 -- c/RConn1
  Three-Phase V-I Measurement3/RConn1 -- Three-Phase Series RLC Branch/LConn1
  Three-Phase Series RLC Branch/LConn2 -- Three-Phase V-I Measurement3/RConn2
  Three-Phase Series RLC Branch/LConn3 -- Three-Phase V-I Measurement3/RConn3
  Three-Phase V-I Measurement3/LConn1 -- Three-Phase V-I Measurement/RConn1
  Three-Phase V-I Measurement3/LConn2 -- Three-Phase V-I Measurement/RConn2
  Three-Phase V-I Measurement3/LConn3 -- Three-Phase V-I Measurement/RConn3
  Ground/LConn1 -- Cf/RConn2 -- Cf/RConn1 -- Cf/RConn3

== system IEEE_39_case3/A3/G4 ==
  Controllers1 : Subsystem  mask{P_set=Pref_sm(4), V_set=Vref_sm(4)}
      mask prompts: P_set "Power Set Point"; V_set "Voltage Set Point"
  Gain1 : Gain  Gain=1/Sb
  Q measurement : Subsystem
  Simplified Synchronous Machine pu Units : spsSimplifiedSynchronousMachinepuUnitsLib/Simplified Synchronous Machine pu Units  ConnectionType=3-wire Y  MechanicalLoad=Mechanical power Pm  MeasurementBus=off  NominalParameters="[ Pn_sm(4)*1e6  Un_sm(4)*1e3  fn_sm(4) ]"  Mechanical=[ H_sm(4) Kd_sm(4) p]  InternalRL="[rs  xd]"  InitialConditions=[dw0_sm theta0_sm ia0_sm ib0_sm ic0_sm pha0_sm phb0_sm phc0_sm]  IterativeDiscreteModel=Trapezoidal non iterative  TsBlock=-1  TsPowergui=0  LoadFlowParameters=[1,0,0,0,0]  Units=0  BusType=PV  Pref=Pref_sm(4)*1e9  Qref=0  Qmin=-inf  Qmax=+inf  PLF=0  QLF=0
      settings: LibrarySourceBlock=|
      | sps_lib/Electrical Machines/Simplified Synchronous
      | Machine pu Units
  A : PMIOPort  Side=Right
  B : PMIOPort  Port=2  Side=Right
  C : PMIOPort  Port=3  Side=Right
  tag scope: Pe4=global, Q4=global, U4=global, theta4=global, w4=global
  wires:
  Controllers1/2(Ef) -> Simplified Synchronous Machine pu Units/2
  Controllers1/1(Pm) -> Simplified Synchronous Machine pu Units/1
  Controllers1/6(Omega) -> [w4]
  Controllers1/4(Uabs) -> [U4]
  Controllers1/5(theta) -> [theta4]
  Controllers1/3(Pe) -> [Pe4]
  Simplified Synchronous Machine pu Units/1 -> Controllers1/1(m)
  [Iabc_33] -> Q measurement/2(Iline)
  Q measurement/1(Q) -> Gain1/1
  [Vabc_33] -> Q measurement/1(Vline)
  Gain1/1 -> [Q4]
  connections:
  A/RConn1 -- Simplified Synchronous Machine pu Units/RConn1
  B/RConn1 -- Simplified Synchronous Machine pu Units/RConn2
  C/RConn1 -- Simplified Synchronous Machine pu Units/RConn3
